simulink model "minhUpdate"  (R2022b)
settings: Solver=VariableStepAuto  StartTime=0.0  StopTime=100  RelTol=1e-3  AbsTol=1e-3  EnableMultiTasking=on
undefined symbols (not defined in the file): h, km, m, s, smiData, X, Y, Z
libraries: sm_lib x316, aerolibconvert2 x25, nesl_utility x22, simulink_extras x9, autolibshared x5, simulink x2, vehdynlibsteering x1
(part 2 of 8)

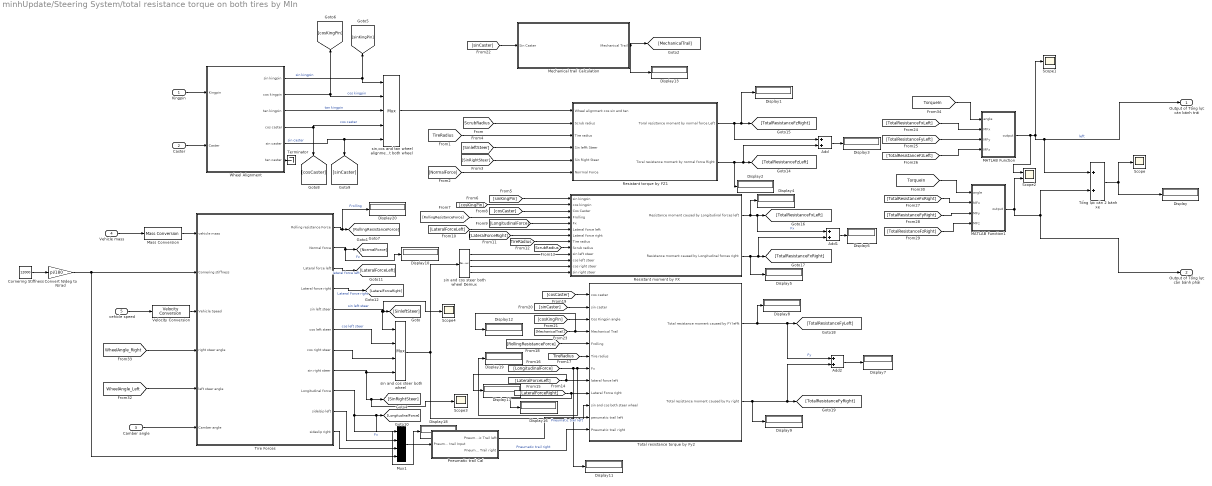
== system minhUpdate/Steering System/total resistance torque on both tires by MIn ==
  Kingpin : Inport
  Caster : Inport  Port=2
  Camber angle : Inport  Port=3
  Vehicle mass : Inport  Port=4
  "vehicle speed " : Inport  Port=5
  Add : Sum
  Add1 : Sum
  Add2 : Sum
  Convert N/deg to N/rad : Gain  Gain=pi/180
  Cornering Stiffness : Constant  Value=12000
  Display{,1..13,16..20} (19 alike) : Display
  MATLAB Function : MATLAB Function  TreatAsAtomicUnit=on
  MATLAB Function1 : MATLAB Function  TreatAsAtomicUnit=on
  Mass Conversion : aerolibconvert2/Mass Conversion  IU=kg  OU=kg
  "Mechanical trail Calculation " : Subsystem
  Mux1 : Mux
  Pneumatic trail Cal : Subsystem
  Resistant moment by FX : Subsystem
  Resistant torque by FZ1 : Subsystem
  Scope{,1,3..4} (4 alike) : Scope
  Scope2 : Scope  NumInputPorts=2
  Terminator : Terminator
  Tire Forces : Subsystem
  Total resistance torque by Fy2 : Subsystem
  Tổng lực cản 2 bánh xe : Sum
  Velocity Conversion : aerolibconvert2/Velocity Conversion  IU=km/h  OU=m/s
  Wheel Alignment : Subsystem
  sin and cos steer both wheel : Mux
  sin and cos steer both wheel Demux : Demux
  sin,cos and tan wheel alignment both wheel : Mux  Inputs=5
  Output of Tổng lực cản bánh trái : Outport
  Output of Tổng lực cản bánh phải : Outport  Port=2
  wires:
  Kingpin/1 -> Wheel Alignment/1(Kingpin)
  Wheel Alignment/6(tan caster) -> Terminator/1
  Vehicle mass/1 -> Mass Conversion/1
  Mass Conversion/1 -> Tire Forces/1(vehicle mass)
  Cornering Stiffness/1 -> Convert N/deg to N/rad/1
  Caster/1 -> Wheel Alignment/2(Caster)
  "vehicle speed "/1 -> Velocity Conversion/1
  [WheelAngle_Right] -> Tire Forces/4("right steer angle ")
  [WheelAngle_Left] -> Tire Forces/5("left steer angle ")
  Velocity Conversion/1 -> Tire Forces/3(Vehicle Speed)
  Tire Forces/11(sideslip right) -> Mux1/3
  Tire Forces/10(sidelsip left) -> Mux1/2
  Tire Forces/9(Longitudinal force) -> Mux1/1, Display18/1, [LongitudinalForce]  "Fx"
  Mux1/1 -> Pneumatic trail Cal/1(Pneumatic trail Input)
  Pneumatic trail Cal/2(Pneumatic Trail right) -> Total resistance torque by Fy2/12(Pneumatic trail right)  "Pneumatic trail right"
  Pneumatic trail Cal/1(Pneumatic Trail left) -> Total resistance torque by Fy2/11(penumatic trail left)  "Pneumatic trail left"
  Tire Forces/5(sin left steer) -> sin and cos steer both wheel/1, Scope4/1, [SinleftSteer]  "sin left steer"
  Tire Forces/6(cos left steer) -> sin and cos steer both wheel/2  "cos left steer"
  Tire Forces/7(cos right steer) -> sin and cos steer both wheel/3
  Tire Forces/8(sin right steer) -> Scope3/1, [SinRightSteer], sin and cos steer both wheel/4
  sin and cos steer both wheel/1 -> Total resistance torque by Fy2/10(sin and cos both steer wheel), sin and cos steer both wheel Demux/1
  Wheel Alignment/1(sin kingpin) -> sin,cos and tan wheel alignment both wheel/1, [sinKingPin]  "sin kingpin"
  Wheel Alignment/2(cos kingpin) -> [cosKingPin], sin,cos and tan wheel alignment both wheel/2  "cos kingpin"
  Wheel Alignment/3(tan kingpin) -> sin,cos and tan wheel alignment both wheel/3  "tan kingpin"
  Wheel Alignment/4(cos caster) -> sin,cos and tan wheel alignment both wheel/4, [cosCaster]  "cos caster"
  Wheel Alignment/5(sin caster) -> [sinCaster], sin,cos and tan wheel alignment both wheel/5  "sin caster"
  sin,cos and tan wheel alignment both wheel/1 -> Resistant torque by FZ1/1("Wheel alignment cos sin and tan ")
  Tire Forces/2(Normal force) -> Display10/1, [NormalForce]  "Fz"
  [ScrubRadius] -> Resistant torque by FZ1/2(Scrub radius)
  [TireRadius] -> Resistant torque by FZ1/3(Tire radius)
  [sinKingPin] -> Resistant moment by FX/1(sin kingpin)
  [cosKingPin] -> Resistant moment by FX/2(cos kingpin)
  Tire Forces/1(Rolling resistance Force) -> Display20/1, [RollingResistanceForce]  "Frolling"
  [RollingResistanceForce] -> Resistant moment by FX/4(Frolling)
  [cosCaster] -> Resistant moment by FX/3(Cos Caster)
  [LongitudinalForce] -> Resistant moment by FX/5(Fx)
  Tire Forces/3(Lateral force left) -> [LateralForceLeft]  "lateral force left"
  Tire Forces/4(Lateral force right) -> [LateralForceRight]  "Lateral Force right"
  [LateralForceLeft] -> Resistant moment by FX/6(Lateral force left)
  [LateralForceRight] -> Resistant moment by FX/7(Lateral force right)
  [TireRadius] -> Resistant moment by FX/8(Tire radius)
  [ScrubRadius] -> Resistant moment by FX/9(Scrub radius)
  [LateralForceRight] -> Display16/1, Total resistance torque by Fy2/9(Lateral Force right)
  [TireRadius] -> Total resistance torque by Fy2/6(Tire radius)
  [RollingResistanceForce] -> Total resistance torque by Fy2/5(Frolling)
  [cosCaster] -> Total resistance torque by Fy2/1(cos caster)
  sin and cos steer both wheel Demux/1 -> Resistant moment by FX/10(sin left steer)
  sin and cos steer both wheel Demux/2 -> Resistant moment by FX/11(cos left steer)
  sin and cos steer both wheel Demux/3 -> Resistant moment by FX/12(cos right steer)
  sin and cos steer both wheel Demux/4 -> Resistant moment by FX/13(sin right steer)
  Resistant moment by FX/1(Resistance moment caused by Longitudinal forces left) -> Display4/1, Add1/1, [TotalResistanceFxLeft]  "Fx"
  Resistant moment by FX/2(Resistance moment caused by Longitudinal forces right) -> Display5/1, Add1/2, [TotalResistanceFxRight]
  Total resistance torque by Fy2/2(Total resistance moment caused by Fy right) -> Display9/1, Add2/2, [TotalResistanceFyRight]
  Total resistance torque by Fy2/1("Total resistance moment caused by FY lefft ") -> Display8/1, Add2/1, [TotalResistanceFyLeft]  "Fy"
  [TotalResistanceFxLeft] -> MATLAB Function/2(MFx)
  [TotalResistanceFyLeft] -> MATLAB Function/3(MFy)
  [TotalResistanceFzLeft] -> MATLAB Function/4(MFz)
  [TotalResistanceFxRight] -> MATLAB Function1/2(MFx)
  [TotalResistanceFyRight] -> MATLAB Function1/3(MFy)
  [TotalResistanceFzRight] -> MATLAB Function1/4(MFz)
  Tổng lực cản 2 bánh xe/1 -> Scope/1, Display/1
  Convert N/deg to N/rad/1 -> Mux1/4, Tire Forces/2(Cornering stiffness)
  [sinCaster] -> Total resistance torque by Fy2/2(sin caster)
  [cosKingPin] -> Total resistance torque by Fy2/3(Cos Kingpin angle)
  [MechanicalTrail] -> Display12/1, Total resistance torque by Fy2/4(Mechanical Trail)
  [LongitudinalForce] -> Display19/1, Total resistance torque by Fy2/7(Fx), Display11/1
  [LateralForceLeft] -> Display17/1, Total resistance torque by Fy2/8(lateral force left)
  [SinleftSteer] -> Resistant torque by FZ1/4(Sin lefft Steer)
  [SinRightSteer] -> Resistant torque by FZ1/5(Sin Right Steer)
  [NormalForce] -> Resistant torque by FZ1/6(Norrmal Force)
  Resistant torque by FZ1/1(Toral resistance moment by normal force Left) -> Add/1, Display1/1, [TotalResistanceFzRight]
  Resistant torque by FZ1/2(Toral resistance moment by normal force Right) -> Display2/1, Add/2, [TotalResistanceFzLeft]
  Add/1 -> Display3/1
  Add1/1 -> Display6/1
  Add2/1 -> Display7/1
  "Mechanical trail Calculation "/1(Mechanical Trail) -> [MechanicalTrail], Display13/1
  [sinCaster] -> "Mechanical trail Calculation "/1(Sin Caster)
  Camber angle/1 -> Tire Forces/6(Camber angle)
  MATLAB Function/1(output) -> Scope2/1, Output of Tổng lực cản bánh trái/1, Tổng lực cản 2 bánh xe/1, Scope1/1  "left"
  [TorqueIn] -> MATLAB Function/1(angle)
  MATLAB Function1/1(output) -> Output of Tổng lực cản bánh phải/1, Tổng lực cản 2 bánh xe/2, Scope2/2
  [TorqueIn] -> MATLAB Function1/1(angle)

== system minhUpdate/total resistance torque on both tires by MIn/Mechanical trail Calculation  ==
  Sin Caster : Inport
  Display{,1..3} (4 alike) : Display
  Divide2 : Product  Inputs=**
  Scrub radius and Tire radius : Subsystem
  Mechanical Trail : Outport
  tag scope: ScrubRadius=global, TireRadius=global
  wires:
  Scrub radius and Tire radius/2(tire radius) -> Divide2/1, Display1/1, [TireRadius]  "Tire radius"
  Sin Caster/1 -> Display2/1, Divide2/2
  Divide2/1 -> Display3/1, Mechanical Trail/1  "Mechanical Trail"
  Scrub radius and Tire radius/1(scrub radius) -> [ScrubRadius], Display/1  "Scub radius"

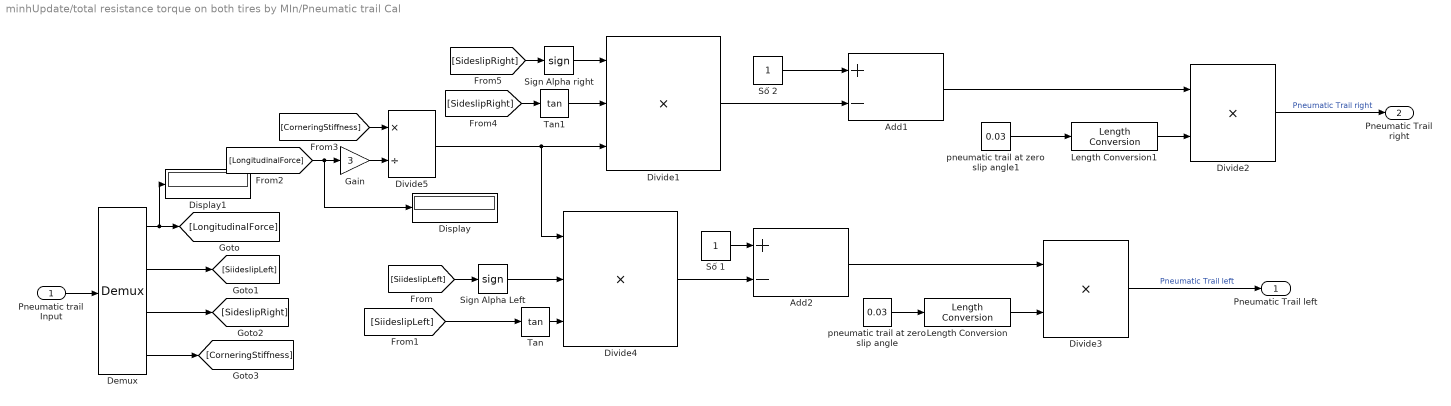
== system minhUpdate/total resistance torque on both tires by MIn/Pneumatic trail Cal ==
  Pneumatic trail Input : Inport
  Add1 : Sum  Inputs=+-
  Add2 : Sum  Inputs=+-
  Demux : Demux
  Display : Display
  Display1 : Display
  Divide1 : Product  Inputs=***
  Divide2 : Product  Inputs=**
  Divide3 : Product  Inputs=**
  Divide4 : Product  Inputs=***
  Divide5 : Product  Inputs=*/
  Gain : Gain  Gain=3
  Length Conversion : aerolibconvert2/Length Conversion  IU=m  OU=m
  Length Conversion1 : aerolibconvert2/Length Conversion  IU=m  OU=m
  Sign Alpha Left : Signum
  Sign Alpha right : Signum
  Số 1 : Constant
  Số 2 : Constant
  Tan : Trigonometry  Operator=tan
  Tan1 : Trigonometry  Operator=tan
  pneumatic trail at zero slip angle : Constant  Value=0.03
  pneumatic trail at zero slip angle1 : Constant  Value=0.03
  Pneumatic Trail left : Outport
  Pneumatic Trail right : Outport  Port=2
  wires:
  Pneumatic trail Input/1 -> Demux/1
  Divide2/1 -> Pneumatic Trail right/1  "Pneumatic Trail right"
  Length Conversion1/1 -> Divide2/2
  Add1/1 -> Divide2/1
  pneumatic trail at zero slip angle1/1 -> Length Conversion1/1
  Số 2/1 -> Add1/1
  Divide1/1 -> Add1/2
  Tan1/1 -> Divide1/2
  Sign Alpha right/1 -> Divide1/1
  Length Conversion/1 -> Divide3/2
  Divide3/1 -> Pneumatic Trail left/1  "Pneumatic Trail left"
  Add2/1 -> Divide3/1
  Gain/1 -> Divide5/2
  pneumatic trail at zero slip angle/1 -> Length Conversion/1
  Tan/1 -> Divide4/3
  Divide5/1 -> Divide4/1, Divide1/3
  Divide4/1 -> Add2/2
  Số 1/1 -> Add2/1
  Sign Alpha Left/1 -> Divide4/2
  Demux/1 -> Display1/1, [LongitudinalForce]
  Demux/2 -> [SiideslipLeft]
  Demux/3 -> [SideslipRight]
  Demux/4 -> [CorneringStiffness]
  [SiideslipLeft] -> Sign Alpha Left/1
  [SiideslipLeft] -> Tan/1
  [SideslipRight] -> Sign Alpha right/1
  [SideslipRight] -> Tan1/1
  [CorneringStiffness] -> Divide5/1
  [LongitudinalForce] -> Display/1, Gain/1

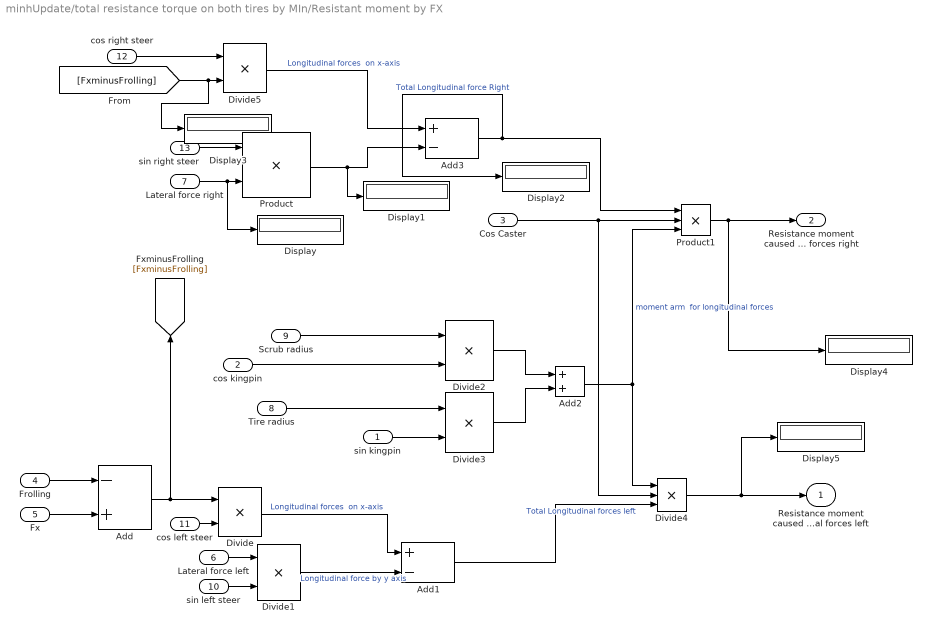
== system minhUpdate/total resistance torque on both tires by MIn/Resistant moment by FX ==
  sin kingpin : Inport
  cos kingpin : Inport  Port=2
  Cos Caster : Inport  Port=3
  Frolling : Inport  Port=4
  Fx : Inport  Port=5
  Lateral force left : Inport  Port=6
  Lateral force right : Inport  Port=7
  Tire radius : Inport  Port=8
  Scrub radius : Inport  Port=9
  sin left steer : Inport  Port=10
  cos left steer : Inport  Port=11
  cos right steer : Inport  Port=12
  sin right steer : Inport  Port=13
  Add : Sum  Inputs=-+
  Add1 : Sum  Inputs=+-
  Add2 : Sum
  Add3 : Sum  Inputs=+-
  Display{,1..5} (6 alike) : Display
  Divide{,1..3,5} (5 alike) : Product  Inputs=**
  Divide4 : Product  Inputs=***
  Product : Product
  Product1 : Product  Inputs=3
  Resistance moment caused by Longitudinal forces left : Outport
  Resistance moment caused by Longitudinal forces right : Outport  Port=2
  wires:
  Scrub radius/1 -> Divide2/1
  Divide/1 -> Add1/1  "Longitudinal forces  on x-axis"
  Divide1/1 -> Add1/2  "Longitudinal force by y axis"
  Lateral force left/1 -> Divide1/1
  Add/1 -> [FxminusFrolling], Divide/1
  Add2/1 -> Divide4/1, Product1/3  "moment arm  for longitudinal forces"
  Divide2/1 -> Add2/1
  Tire radius/1 -> Divide3/1
  Divide3/1 -> Add2/2
  cos kingpin/1 -> Divide2/2
  cos left steer/1 -> Divide/2
  sin left steer/1 -> Divide1/2
  Fx/1 -> Add/2
  Frolling/1 -> Add/1
  sin kingpin/1 -> Divide3/2
  Lateral force right/1 -> Display/1, Product/2
  sin right steer/1 -> Product/1
  Product/1 -> Display1/1, Add3/2
  cos right steer/1 -> Divide5/1
  Divide5/1 -> Add3/1  "Longitudinal forces  on x-axis"
  Add3/1 -> Display2/1, Product1/1  "Total Longitudinal force Right"
  Divide4/1 -> Display5/1, Resistance moment caused by Longitudinal forces left/1
  Cos Caster/1 -> Product1/2, Divide4/2
  Product1/1 -> Resistance moment caused by Longitudinal forces right/1, Display4/1
  [FxminusFrolling] -> Display3/1, Divide5/2
  Add1/1 -> Divide4/3  "Total Longitudinal forces left"

== system minhUpdate/total resistance torque on both tires by MIn/Resistant torque by FZ1 ==
  "Wheel alignment cos sin and tan " : Inport
  Scrub radius : Inport  Port=2
  Tire radius : Inport  Port=3
  Sin lefft Steer : Inport  Port=4
  Sin Right Steer : Inport  Port=5
  Norrmal Force : Inport  Port=6
  Add : Sum
  Demux : Demux  Outputs=5
  Display{,1..4} (5 alike) : Display
  Divide{,1..3} (4 alike) : Product  Inputs=**
  Terminator : Terminator
  Total Normal force Right : Product  Inputs=****
  Total Normal force left : Product  Inputs=****
  Toral resistance moment by normal force Left : Outport
  Toral resistance moment by normal force Right : Outport  Port=2
  wires:
  Tire radius/1 -> Divide/1
  Scrub radius/1 -> Add/1
  Total Normal force left/1 -> Divide2/2, Display1/1  "Normal force left"
  Divide1/1 -> Divide3/1, Divide2/1  "moment arm of Fz"
  Divide/1 -> Add/2
  Add/1 -> Divide1/1
  Sin lefft Steer/1 -> Display2/1, Total Normal force left/3
  Demux/3 -> Divide/2  "tan kingpin"
  Divide2/1 -> Toral resistance moment by normal force Left/1
  Demux/5 -> Terminator/1
  "Wheel alignment cos sin and tan "/1 -> Demux/1
  Sin Right Steer/1 -> Total Normal force Right/3
  Norrmal Force/1 -> Display/1, Total Normal force left/4, Total Normal force Right/4
  Total Normal force Right/1 -> Divide3/2  "Normal force right"
  Divide3/1 -> Toral resistance moment by normal force Right/1
  Demux/1 -> [sinKingpin]  "sin kingppin"
  Demux/2 -> [cosKingpin]  "cos kingpin"
  Demux/4 -> [cosCaster]  "cos caster"
  [cosKingpin] -> Divide1/2
  [cosCaster] -> Total Normal force Right/2
  [sinKingpin] -> Total Normal force Right/1
  [sinKingpin] -> Display3/1, Total Normal force left/1
  [cosCaster] -> Display4/1, Total Normal force left/2

== system minhUpdate/total resistance torque on both tires by MIn/Tire Forces ==
  vehicle mass : Inport
  Cornering stiffness : Inport  Port=2
  Vehicle Speed : Inport  Port=3
  "right steer angle " : Inport  Port=4
  "left steer angle " : Inport  Port=5
  Camber angle : Inport  Port=6
  Add : Sum
  Add1 : Sum
  Cos : Trigonometry  Operator=cos
  Cos1 : Trigonometry  Operator=cos
  Display{,1..4} (5 alike) : Display
  Lateral Force Area : Subsystem
  Mass Conversion : aerolibconvert2/Mass Conversion  IU=kg  OU=kg
  Multiply : Gain  Gain=130
  Normal and Longitudinal force Area : Subsystem
  Rolling Resistance area : Subsystem
  Sin1 : Trigonometry
  Sin2 : Trigonometry
  Rolling resistance Force : Outport
  Normal force : Outport  Port=2
  Lateral force left : Outport  Port=3
  Lateral force right : Outport  Port=4
  sin left steer : Outport  Port=5
  cos left steer : Outport  Port=6
  cos right steer : Outport  Port=7
  sin right steer : Outport  Port=8
  Longitudinal force : Outport  Port=9
  sidelsip left : Outport  Port=10
  sideslip right : Outport  Port=11
  wires:
  Lateral Force Area/4(Right Steer angle) -> Sin2/1, Cos1/1
  vehicle mass/1 -> Display/1, Mass Conversion/1
  Sin2/1 -> sin right steer/1  "sin right  steer"
  Cos1/1 -> cos right steer/1  "cos right steer"
  Normal and Longitudinal force Area/1(Longitudinal force) -> Longitudinal force/1
  Normal and Longitudinal force Area/2(Normal force) -> Normal force/1
  Rolling Resistance area/1(rolling resitance force) -> Rolling resistance Force/1  "Rolling resistance Force"
  Lateral Force Area/5(sideslip left) -> sidelsip left/1
  Lateral Force Area/6("sideslip right ") -> sideslip right/1
  Cornering stiffness/1 -> Lateral Force Area/1("Cornering Stiffness ")
  Mass Conversion/1 -> Display1/1, Normal and Longitudinal force Area/1(vehicle mass), Display2/1, Rolling Resistance area/1(vehicle mass)
  Vehicle Speed/1 -> Lateral Force Area/2(Vehicle Speed)
  "left steer angle "/1 -> Lateral Force Area/4(Steering angle from left)
  "right steer angle "/1 -> Lateral Force Area/3(Steering angle right)
  Lateral Force Area/3(Left steer angle) -> Sin1/1, Cos/1
  Sin1/1 -> sin left steer/1  "sin left  steer"
  Cos/1 -> cos left steer/1  "cos left steer"
  Camber angle/1 -> Multiply/1
  Multiply/1 -> Add1/1, Add/1
  Lateral Force Area/1(Lateral force left(N)) -> Add/2
  Lateral Force Area/2("Lateral force right(N)  ") -> Add1/2
  Add1/1 -> Display4/1, Lateral force right/1
  Add/1 -> Display3/1, Lateral force left/1

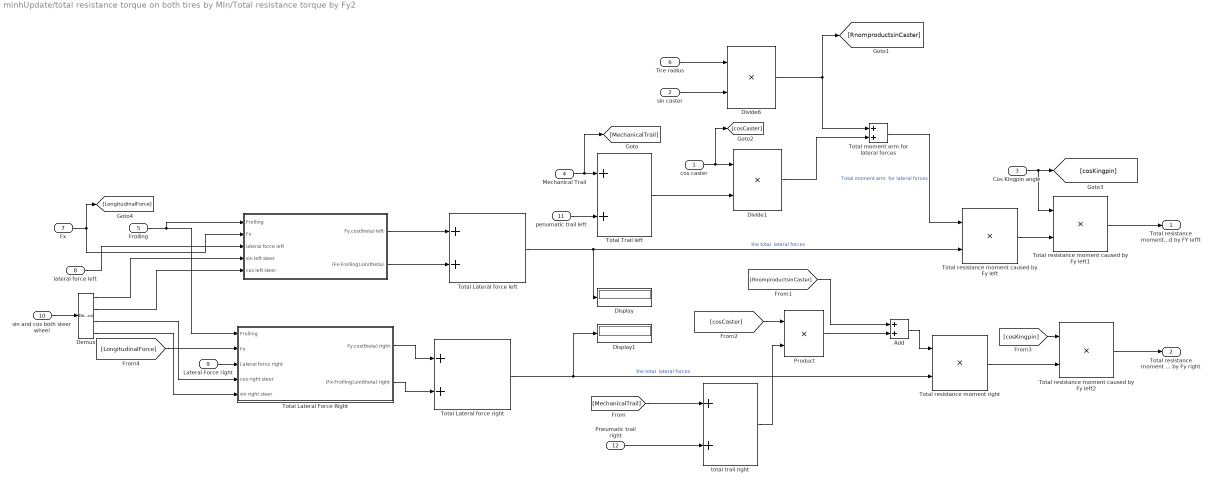
== system minhUpdate/total resistance torque on both tires by MIn/Total resistance torque by Fy2 ==
  cos caster : Inport
  sin caster : Inport  Port=2
  Cos Kingpin angle : Inport  Port=3
  Mechanical Trail : Inport  Port=4
  Frolling : Inport  Port=5
  Tire radius : Inport  Port=6
  Fx : Inport  Port=7
  lateral force left : Inport  Port=8
  Lateral Force right : Inport  Port=9
  sin and cos both steer wheel : Inport  Port=10
  penumatic trail left : Inport  Port=11
  Pneumatic trail right : Inport  Port=12
  " " : Subsystem
  " Total Lateral Force Right " : Subsystem
  Add : Sum
  Demux : Demux
  Display : Display
  Display1 : Display
  Divide1 : Product  Inputs=**
  Divide6 : Product  Inputs=**
  Product : Product
  Total Lateral force left : Sum
  Total Lateral force right : Sum
  Total Trail left : Sum
  Total moment arm for lateral forces : Sum
  Total resistance moment caused by Fy left : Product  Inputs=**
  Total resistance moment caused by Fy left1 : Product  Inputs=**
  Total resistance moment caused by Fy left2 : Product  Inputs=**
  Total resistance moment right : Product  Inputs=**
  total trail right : Sum
  "Total resistance moment caused by FY lefft " : Outport
  Total resistance moment caused by Fy right : Outport  Port=2
  wires:
  cos caster/1 -> [cosCaster], Divide1/1
  Divide6/1 -> [RnomproductsinCaster], Total moment arm for lateral forces/1
  Total moment arm for lateral forces/1 -> Total resistance moment caused by Fy left/1  "Total moment arm  for lateral forces"
  Total Lateral force left/1 -> Display/1, Total resistance moment caused by Fy left/2  "the total  lateral forces"
  Divide1/1 -> Total moment arm for lateral forces/2
  " "/1(Fy.cos(theta) left) -> Total Lateral force left/1
  Total Trail left/1 -> Divide1/2
  " "/2((Fx-Frolling).sin(theta)) -> Total Lateral force left/2
  penumatic trail left/1 -> Total Trail left/2
  Tire radius/1 -> Divide6/1
  sin caster/1 -> Divide6/2
  Frolling/1 -> " Total Lateral Force Right "/1(Frolling), " "/1(Frolling)
  lateral force left/1 -> " "/3(lateral force left)
  Mechanical Trail/1 -> [MechanicalTrail], Total Trail left/1
  Lateral Force right/1 -> " Total Lateral Force Right "/3(Lateral force right)
  Demux/3 -> " Total Lateral Force Right "/4(cos right steer)
  Demux/4 -> " Total Lateral Force Right "/5(sin right steer)
  " Total Lateral Force Right "/1(Fy.cos(theta) right) -> Total Lateral force right/1
  " Total Lateral Force Right "/2((Fx-Frolling).sin(theta) right) -> Total Lateral force right/2
  Total Lateral force right/1 -> Display1/1, Total resistance moment right/2  "the total  lateral forces"
  Cos Kingpin angle/1 -> [cosKingpin], Total resistance moment caused by Fy left1/1
  Total resistance moment caused by Fy left/1 -> Total resistance moment caused by Fy left1/2
  Total resistance moment caused by Fy left1/1 -> "Total resistance moment caused by FY lefft "/1
  Total resistance moment right/1 -> Total resistance moment caused by Fy left2/2
  Total resistance moment caused by Fy left2/1 -> Total resistance moment caused by Fy right/1
  Pneumatic trail right/1 -> total trail right/2
  total trail right/1 -> Product/2
  Product/1 -> Add/2
  Add/1 -> Total resistance moment right/1
  Demux/1 -> " "/4(sin left steer)
  Demux/2 -> " "/5(cos left steer)
  sin and cos both steer wheel/1 -> Demux/1
  [MechanicalTrail] -> total trail right/1
  [RnomproductsinCaster] -> Add/1
  [cosCaster] -> Product/1
  [cosKingpin] -> Total resistance moment caused by Fy left2/1
  Fx/1 -> " "/2(Fx), [LongitudinalForce]
  [LongitudinalForce] -> " Total Lateral Force Right "/2(Fx)

== system minhUpdate/total resistance torque on both tires by MIn/Wheel Alignment ==
  Kingpin : Inport
  Caster : Inport  Port=2
  Cos : Trigonometry  Operator=cos
  Cos1 : Trigonometry  Operator=cos
  Degrees to Radians : simulink_extras/Transformations/Degrees to Radians
  Degrees to Radians1 : simulink_extras/Transformations/Degrees to Radians
  Display : Display
  Sin : Trigonometry
  Sin1 : Trigonometry
  Tan : Trigonometry  Operator=tan
  Tan1 : Trigonometry  Operator=tan
  sin kingpin : Outport
  cos kingpin : Outport  Port=2
  tan kingpin : Outport  Port=3
  cos caster : Outport  Port=4
  sin caster : Outport  Port=5
  tan caster : Outport  Port=6
  wires:
  Sin1/1 -> sin caster/1
  Degrees to Radians1/1 -> Tan1/1, Sin1/1, Cos1/1
  Sin/1 -> sin kingpin/1
  Caster/1 -> Degrees to Radians1/1
  Cos1/1 -> cos caster/1
  Cos/1 -> cos kingpin/1
  Degrees to Radians/1 -> Tan/1, Sin/1, Cos/1
  Kingpin/1 -> Degrees to Radians/1
  Tan/1 -> Display/1, tan kingpin/1
  Tan1/1 -> tan caster/1

== system minhUpdate/Steering System/Chassis + Rack/Rack Case + Chassis ==
  PS-Simulink Converter : nesl_utility/PS-Simulink Converter  PhysicalDomain=network_engine_domain  SubClassName=ps_output  LeftPortType=input  RightPortType=output  PseudoPeriodic=off  Frequencies=[]  VectorFormat=1-D array  Unit=inherit  AffineConversion=off
  PS-Simulink Converter1 : nesl_utility/PS-Simulink Converter  PhysicalDomain=network_engine_domain  SubClassName=ps_output  LeftPortType=input  RightPortType=output  PseudoPeriodic=off  Frequencies=[]  VectorFormat=1-D array  Unit=inherit  AffineConversion=off
  Parallel : sm_lib/Constraints/Angle Constraint  ConstraintType=Parallel  Angle=45  AngleUnits=deg  SenseSignedTorqueMagnitude=off  SenseTorque=off  SenseForce=off  WrenchDir=FollowerOnBase  WrenchFrame=BaseFrame
  Parallel1 : sm_lib/Constraints/Angle Constraint  ConstraintType=Parallel  Angle=45  AngleUnits=deg  SenseSignedTorqueMagnitude=off  SenseTorque=off  SenseForce=off  WrenchDir=FollowerOnBase  WrenchFrame=BaseFrame
  Prismatic Joint : sm_lib/Joints/Prismatic Joint  JointMode=Normal  SenseConstraintForce=off  SenseConstraintForceX=off  SenseConstraintForceY=off  SenseConstraintForceZ=off  SenseConstraintTorque=off  SenseConstraintTorqueX=off  SenseConstraintTorqueY=off  SenseConstraintTorqueZ=off  SenseTotalForce=off  SenseTotalForceX=off  SenseTotalForceY=off  SenseTotalForceZ=off  SenseTotalTorque=off  SenseTotalTorqueX=off  SenseTotalTorqueY=off  SenseTotalTorqueZ=off  CompositeWrenchDir=FollowerOnBase  CompositeWrenchFrame=BaseFrame  EquilibriumPosition=0  EquilibriumPositionUnits=m  SpringStiffness=0  SpringStiffnessUnits=N/m  DampingCoefficient=0  DampingCoefficientUnits=N/(m/s)  TorqueActuationMode=NoTorque  MotionActuationMode=ComputedMotion  SensePosition=off  SenseVelocity=off  SenseAcceleration=off  SenseTorqueForce=off  SenseLowerLimitTorqueForce=off  SenseUpperLimitTorqueForce=off  LowerLimitSpecify=off  LowerLimitBound=-1  LowerLimitBoundUnits=m  LowerLimitStiffness=1e6  LowerLimitStiffnessUnits=N/m  LowerLimitDamping=1e3  LowerLimitDampingUnits=N/(m/s)  LowerLimitTransitionRegionWidth=1e-4  LowerLimitTransitionRegionWidthUnits=m  UpperLimitSpecify=off  UpperLimitBound=1  UpperLimitBoundUnits=m  UpperLimitStiffness=1e6  UpperLimitStiffnessUnits=N/m  UpperLimitDamping=1e3  UpperLimitDampingUnits=N/(m/s)  UpperLimitTransitionRegionWidth=1e-4  UpperLimitTransitionRegionWidthUnits=m  PositionTargetSpecify=off  PositionTargetPriority=High  PositionTargetValue=0  PositionTargetValueUnits=m  VelocityTargetSpecify=off  VelocityTargetPriority=High  VelocityTargetValue=0  VelocityTargetValueUnits=m/s
  Rack_housing_1_RIGID : Subsystem
  Revolute Joint : sm_lib/Joints/Revolute Joint  JointMode=Normal  SenseConstraintForce=off  SenseConstraintForceX=off  SenseConstraintForceY=off  SenseConstraintForceZ=off  SenseConstraintTorque=off  SenseConstraintTorqueX=off  SenseConstraintTorqueY=off  SenseConstraintTorqueZ=off  SenseTotalForce=off  SenseTotalForceX=off  SenseTotalForceY=off  SenseTotalForceZ=off  SenseTotalTorque=off  SenseTotalTorqueX=off  SenseTotalTorqueY=off  SenseTotalTorqueZ=off  CompositeWrenchDir=FollowerOnBase  CompositeWrenchFrame=BaseFrame  EquilibriumPosition=0  EquilibriumPositionUnits=deg  SpringStiffness=0  SpringStiffnessUnits=N*m/rad  DampingCoefficient=8  DampingCoefficientUnits=N*m/(rad/s)  TorqueActuationMode=NoTorque  MotionActuationMode=ComputedMotion  SensePosition=on  SenseVelocity=on  SenseAcceleration=off  SenseTorqueForce=off  SenseLowerLimitTorqueForce=off  SenseUpperLimitTorqueForce=off  LowerLimitSpecify=off  LowerLimitBound=-90  LowerLimitBoundUnits=deg  LowerLimitStiffness=1e4  LowerLimitStiffnessUnits=N*m/deg  LowerLimitDamping=10  LowerLimitDampingUnits=N*m/(deg/s)  LowerLimitTransitionRegionWidth=0.1  LowerLimitTransitionRegionWidthUnits=deg  UpperLimitSpecify=off  UpperLimitBound=90  UpperLimitBoundUnits=deg  UpperLimitStiffness=1e4  UpperLimitStiffnessUnits=N*m/deg  UpperLimitDamping=10  UpperLimitDampingUnits=N*m/(deg/s)  UpperLimitTransitionRegionWidth=0.1  UpperLimitTransitionRegionWidthUnits=deg  PositionTargetSpecify=off  PositionTargetPriority=High  PositionTargetValue=0  PositionTargetValueUnits=deg  VelocityTargetSpecify=on  VelocityTargetPriority=High  VelocityTargetValue=0  VelocityTargetValueUnits=deg/s
  Revolute4 : sm_lib/Joints/Revolute Joint  JointMode=Normal  SenseConstraintForce=off  SenseConstraintForceX=off  SenseConstraintForceY=off  SenseConstraintForceZ=off  SenseConstraintTorque=off  SenseConstraintTorqueX=off  SenseConstraintTorqueY=off  SenseConstraintTorqueZ=off  SenseTotalForce=off  SenseTotalForceX=off  SenseTotalForceY=off  SenseTotalForceZ=off  SenseTotalTorque=off  SenseTotalTorqueX=off  SenseTotalTorqueY=off  SenseTotalTorqueZ=off  CompositeWrenchDir=FollowerOnBase  CompositeWrenchFrame=BaseFrame  EquilibriumPosition=0  EquilibriumPositionUnits=deg  SpringStiffness=0  SpringStiffnessUnits=N*m/deg  DampingCoefficient=0  DampingCoefficientUnits=N*m/(deg/s)  TorqueActuationMode=NoTorque  MotionActuationMode=ComputedMotion  SensePosition=off  SenseVelocity=off  SenseAcceleration=off  SenseTorqueForce=off  SenseLowerLimitTorqueForce=off  SenseUpperLimitTorqueForce=off  LowerLimitSpecify=off  LowerLimitBound=-90  LowerLimitBoundUnits=deg  LowerLimitStiffness=1e4  LowerLimitStiffnessUnits=N*m/deg  LowerLimitDamping=10  LowerLimitDampingUnits=N*m/(deg/s)  LowerLimitTransitionRegionWidth=0.1  LowerLimitTransitionRegionWidthUnits=deg  UpperLimitSpecify=off  UpperLimitBound=90  UpperLimitBoundUnits=deg  UpperLimitStiffness=1e4  UpperLimitStiffnessUnits=N*m/deg  UpperLimitDamping=10  UpperLimitDampingUnits=N*m/(deg/s)  UpperLimitTransitionRegionWidth=0.1  UpperLimitTransitionRegionWidthUnits=deg  PositionTargetSpecify=on  PositionTargetPriority=Low  PositionTargetValue=smiData.RevoluteJoint(5).Rz.Pos  PositionTargetValueUnits=deg  VelocityTargetSpecify=off  VelocityTargetPriority=High  VelocityTargetValue=0  VelocityTargetValueUnits=deg/s
  Revolute5 : sm_lib/Joints/Revolute Joint  JointMode=Normal  SenseConstraintForce=off  SenseConstraintForceX=off  SenseConstraintForceY=off  SenseConstraintForceZ=off  SenseConstraintTorque=off  SenseConstraintTorqueX=off  SenseConstraintTorqueY=off  SenseConstraintTorqueZ=off  SenseTotalForce=off  SenseTotalForceX=off  SenseTotalForceY=off  SenseTotalForceZ=off  SenseTotalTorque=off  SenseTotalTorqueX=off  SenseTotalTorqueY=off  SenseTotalTorqueZ=off  CompositeWrenchDir=FollowerOnBase  CompositeWrenchFrame=BaseFrame  EquilibriumPosition=0  EquilibriumPositionUnits=deg  SpringStiffness=0  SpringStiffnessUnits=N*m/deg  DampingCoefficient=0  DampingCoefficientUnits=N*m/(deg/s)  TorqueActuationMode=NoTorque  MotionActuationMode=ComputedMotion  SensePosition=off  SenseVelocity=off  SenseAcceleration=off  SenseTorqueForce=off  SenseLowerLimitTorqueForce=off  SenseUpperLimitTorqueForce=off  LowerLimitSpecify=off  LowerLimitBound=-90  LowerLimitBoundUnits=deg  LowerLimitStiffness=1e4  LowerLimitStiffnessUnits=N*m/deg  LowerLimitDamping=10  LowerLimitDampingUnits=N*m/(deg/s)  LowerLimitTransitionRegionWidth=0.1  LowerLimitTransitionRegionWidthUnits=deg  UpperLimitSpecify=off  UpperLimitBound=90  UpperLimitBoundUnits=deg  UpperLimitStiffness=1e4  UpperLimitStiffnessUnits=N*m/deg  UpperLimitDamping=10  UpperLimitDampingUnits=N*m/(deg/s)  UpperLimitTransitionRegionWidth=0.1  UpperLimitTransitionRegionWidthUnits=deg  PositionTargetSpecify=on  PositionTargetPriority=Low  PositionTargetValue=smiData.RevoluteJoint(6).Rz.Pos  PositionTargetValueUnits=deg  VelocityTargetSpecify=off  VelocityTargetPriority=High  VelocityTargetValue=0  VelocityTargetValueUnits=deg/s
  Revolute6 : sm_lib/Joints/Revolute Joint  JointMode=Normal  SenseConstraintForce=off  SenseConstraintForceX=off  SenseConstraintForceY=off  SenseConstraintForceZ=off  SenseConstraintTorque=off  SenseConstraintTorqueX=off  SenseConstraintTorqueY=off  SenseConstraintTorqueZ=off  SenseTotalForce=off  SenseTotalForceX=off  SenseTotalForceY=off  SenseTotalForceZ=off  SenseTotalTorque=off  SenseTotalTorqueX=off  SenseTotalTorqueY=off  SenseTotalTorqueZ=off  CompositeWrenchDir=FollowerOnBase  CompositeWrenchFrame=BaseFrame  EquilibriumPosition=0  EquilibriumPositionUnits=deg  SpringStiffness=0  SpringStiffnessUnits=N*m/deg  DampingCoefficient=0  DampingCoefficientUnits=N*m/(deg/s)  TorqueActuationMode=NoTorque  MotionActuationMode=ComputedMotion  SensePosition=off  SenseVelocity=off  SenseAcceleration=off  SenseTorqueForce=off  SenseLowerLimitTorqueForce=off  SenseUpperLimitTorqueForce=off  LowerLimitSpecify=off  LowerLimitBound=-90  LowerLimitBoundUnits=deg  LowerLimitStiffness=1e4  LowerLimitStiffnessUnits=N*m/deg  LowerLimitDamping=10  LowerLimitDampingUnits=N*m/(deg/s)  LowerLimitTransitionRegionWidth=0.1  LowerLimitTransitionRegionWidthUnits=deg  UpperLimitSpecify=off  UpperLimitBound=90  UpperLimitBoundUnits=deg  UpperLimitStiffness=1e4  UpperLimitStiffnessUnits=N*m/deg  UpperLimitDamping=10  UpperLimitDampingUnits=N*m/(deg/s)  UpperLimitTransitionRegionWidth=0.1  UpperLimitTransitionRegionWidthUnits=deg  PositionTargetSpecify=on  PositionTargetPriority=Low  PositionTargetValue=smiData.RevoluteJoint(7).Rz.Pos  PositionTargetValueUnits=deg  VelocityTargetSpecify=off  VelocityTargetPriority=High  VelocityTargetValue=0  VelocityTargetValueUnits=deg/s
  Revolute7 : sm_lib/Joints/Revolute Joint  JointMode=Normal  SenseConstraintForce=off  SenseConstraintForceX=off  SenseConstraintForceY=off  SenseConstraintForceZ=off  SenseConstraintTorque=off  SenseConstraintTorqueX=off  SenseConstraintTorqueY=off  SenseConstraintTorqueZ=off  SenseTotalForce=off  SenseTotalForceX=off  SenseTotalForceY=off  SenseTotalForceZ=off  SenseTotalTorque=off  SenseTotalTorqueX=off  SenseTotalTorqueY=off  SenseTotalTorqueZ=off  CompositeWrenchDir=FollowerOnBase  CompositeWrenchFrame=BaseFrame  EquilibriumPosition=0  EquilibriumPositionUnits=deg  SpringStiffness=0  SpringStiffnessUnits=N*m/deg  DampingCoefficient=0  DampingCoefficientUnits=N*m/(deg/s)  TorqueActuationMode=NoTorque  MotionActuationMode=ComputedMotion  SensePosition=off  SenseVelocity=off  SenseAcceleration=off  SenseTorqueForce=off  SenseLowerLimitTorqueForce=off  SenseUpperLimitTorqueForce=off  LowerLimitSpecify=off  LowerLimitBound=-90  LowerLimitBoundUnits=deg  LowerLimitStiffness=1e4  LowerLimitStiffnessUnits=N*m/deg  LowerLimitDamping=10  LowerLimitDampingUnits=N*m/(deg/s)  LowerLimitTransitionRegionWidth=0.1  LowerLimitTransitionRegionWidthUnits=deg  UpperLimitSpecify=off  UpperLimitBound=90  UpperLimitBoundUnits=deg  UpperLimitStiffness=1e4  UpperLimitStiffnessUnits=N*m/deg  UpperLimitDamping=10  UpperLimitDampingUnits=N*m/(deg/s)  UpperLimitTransitionRegionWidth=0.1  UpperLimitTransitionRegionWidthUnits=deg  PositionTargetSpecify=on  PositionTargetPriority=Low  PositionTargetValue=smiData.RevoluteJoint(8).Rz.Pos  PositionTargetValueUnits=deg  VelocityTargetSpecify=off  VelocityTargetPriority=High  VelocityTargetValue=0  VelocityTargetValueUnits=deg/s
  Revolute8 : sm_lib/Joints/Revolute Joint  JointMode=Normal  SenseConstraintForce=off  SenseConstraintForceX=off  SenseConstraintForceY=off  SenseConstraintForceZ=off  SenseConstraintTorque=off  SenseConstraintTorqueX=off  SenseConstraintTorqueY=off  SenseConstraintTorqueZ=off  SenseTotalForce=off  SenseTotalForceX=off  SenseTotalForceY=off  SenseTotalForceZ=off  SenseTotalTorque=off  SenseTotalTorqueX=off  SenseTotalTorqueY=off  SenseTotalTorqueZ=off  CompositeWrenchDir=FollowerOnBase  CompositeWrenchFrame=BaseFrame  EquilibriumPosition=0  EquilibriumPositionUnits=deg  SpringStiffness=0  SpringStiffnessUnits=N*m/deg  DampingCoefficient=0  DampingCoefficientUnits=N*m/(deg/s)  TorqueActuationMode=NoTorque  MotionActuationMode=ComputedMotion  SensePosition=off  SenseVelocity=off  SenseAcceleration=off  SenseTorqueForce=off  SenseLowerLimitTorqueForce=off  SenseUpperLimitTorqueForce=off  LowerLimitSpecify=off  LowerLimitBound=-90  LowerLimitBoundUnits=deg  LowerLimitStiffness=1e4  LowerLimitStiffnessUnits=N*m/deg  LowerLimitDamping=10  LowerLimitDampingUnits=N*m/(deg/s)  LowerLimitTransitionRegionWidth=0.1  LowerLimitTransitionRegionWidthUnits=deg  UpperLimitSpecify=off  UpperLimitBound=90  UpperLimitBoundUnits=deg  UpperLimitStiffness=1e4  UpperLimitStiffnessUnits=N*m/deg  UpperLimitDamping=10  UpperLimitDampingUnits=N*m/(deg/s)  UpperLimitTransitionRegionWidth=0.1  UpperLimitTransitionRegionWidthUnits=deg  PositionTargetSpecify=on  PositionTargetPriority=Low  PositionTargetValue=smiData.RevoluteJoint(9).Rz.Pos  PositionTargetValueUnits=deg  VelocityTargetSpecify=off  VelocityTargetPriority=High  VelocityTargetValue=0  VelocityTargetValueUnits=deg/s
  Revolute9 : sm_lib/Joints/Revolute Joint  JointMode=Normal  SenseConstraintForce=off  SenseConstraintForceX=off  SenseConstraintForceY=off  SenseConstraintForceZ=off  SenseConstraintTorque=off  SenseConstraintTorqueX=off  SenseConstraintTorqueY=off  SenseConstraintTorqueZ=off  SenseTotalForce=off  SenseTotalForceX=off  SenseTotalForceY=off  SenseTotalForceZ=off  SenseTotalTorque=off  SenseTotalTorqueX=off  SenseTotalTorqueY=off  SenseTotalTorqueZ=off  CompositeWrenchDir=FollowerOnBase  CompositeWrenchFrame=BaseFrame  EquilibriumPosition=0  EquilibriumPositionUnits=deg  SpringStiffness=0  SpringStiffnessUnits=N*m/deg  DampingCoefficient=0  DampingCoefficientUnits=N*m/(deg/s)  TorqueActuationMode=NoTorque  MotionActuationMode=ComputedMotion  SensePosition=off  SenseVelocity=off  SenseAcceleration=off  SenseTorqueForce=off  SenseLowerLimitTorqueForce=off  SenseUpperLimitTorqueForce=off  LowerLimitSpecify=off  LowerLimitBound=-90  LowerLimitBoundUnits=deg  LowerLimitStiffness=1e4  LowerLimitStiffnessUnits=N*m/deg  LowerLimitDamping=10  LowerLimitDampingUnits=N*m/(deg/s)  LowerLimitTransitionRegionWidth=0.1  LowerLimitTransitionRegionWidthUnits=deg  UpperLimitSpecify=off  UpperLimitBound=90  UpperLimitBoundUnits=deg  UpperLimitStiffness=1e4  UpperLimitStiffnessUnits=N*m/deg  UpperLimitDamping=10  UpperLimitDampingUnits=N*m/(deg/s)  UpperLimitTransitionRegionWidth=0.1  UpperLimitTransitionRegionWidthUnits=deg  PositionTargetSpecify=off  PositionTargetPriority=High  PositionTargetValue=0  PositionTargetValueUnits=deg  VelocityTargetSpecify=off  VelocityTargetPriority=High  VelocityTargetValue=0  VelocityTargetValueUnits=deg/s
  Transform : sm_lib/Frames and Transforms/Rigid Transform  TranslationMethod=Cartesian  TranslationStandardOffset=0  TranslationLengthUnit=mm  TranslationStandardAxis=+Z  TranslationCartesianOffset=smiData.RigidTransform(47).translation  TranslationROffset=0  TranslationROffsetUnits=m  TranslationZOffset=0  TranslationZOffsetUnits=m  TranslationThetaOffset=0  TranslationThetaOffsetUnits=deg  RotationMethod=ArbitraryAxis  RotationAngleUnits=rad  RotationStandardAxis=+Z  RotationAngle=smiData.RigidTransform(47).angle  RotationArbitraryAxis=smiData.RigidTransform(47).axis  FollAlignAxisA=+X  BaseAlignAxisA=+Y  FollAlignAxisB=+Y  BaseAlignAxisB=+Z  RotationSequenceAxes=FollowerAxes  RotationSequence=XYX  RotationSequenceAngles=[0 0 0]  RotationSequenceAnglesUnits=deg  RotationMatrix=[1 0 0; 0 1 0; 0 0 1]  Quaternion=[1 0 0 0]
  extention_rod_1_RIGID : Subsystem
  extention_rod_2_RIGID : Subsystem
  extention_rod_image_1_RIGID : Subsystem
  extention_rod_image_2_RIGID : Subsystem
  lever_arm_by_Long_1_RIGID : Subsystem
  lever_arm_by_Long_2_RIGID : Subsystem
  lever_arm_mini_by_Long_1_RIGID : Subsystem
  lever_arm_mini_by_Long_2_RIGID : Subsystem
  Conn1 : PMIOPort  Side=Left
  Conn3 : PMIOPort  Port=2  Side=Left
  Conn4 : PMIOPort  Port=3  Side=Left
  Conn5 : PMIOPort  Port=4  Side=Left
  F : PMIOPort  Port=5  Side=Left
  F1 : PMIOPort  Port=6  Side=Left
  F2 : PMIOPort  Port=7  Side=Left
  Conn2 : PMIOPort  Port=8  Side=Right
  F3 : PMIOPort  Port=9  Side=Right
  Steering Wheel Angle : Outport
  Steering Wheel Velocity : Outport  Port=2
  wires:
  PS-Simulink Converter/1 -> Steering Wheel Angle/1
  PS-Simulink Converter1/1 -> Steering Wheel Velocity/1
  connections:
  Parallel/RConn1 -- extention_rod_1_RIGID/LConn1
  Revolute Joint/RConn1 -- Rack_housing_1_RIGID/LConn2
  Revolute8/LConn1 -- lever_arm_by_Long_2_RIGID/RConn1
  Parallel/LConn1 -- Rack_housing_1_RIGID/RConn2
  Parallel1/LConn1 -- Rack_housing_1_RIGID/RConn1
  F/RConn1 -- extention_rod_image_2_RIGID/LConn1
  Rack_housing_1_RIGID/LConn1 -- Transform/RConn1
  Parallel1/RConn1 -- extention_rod_2_RIGID/LConn1
  Revolute6/RConn1 -- lever_arm_mini_by_Long_1_RIGID/LConn1
  Revolute4/RConn1 -- extention_rod_1_RIGID/LConn2
  Revolute7/RConn1 -- lever_arm_by_Long_1_RIGID/LConn1
  Revolute9/RConn1 -- lever_arm_by_Long_2_RIGID/LConn1
  Revolute6/LConn1 -- lever_arm_by_Long_1_RIGID/RConn1
  Revolute7/LConn1 -- extention_rod_1_RIGID/RConn1
  Revolute5/RConn1 -- extention_rod_2_RIGID/LConn2
  Prismatic Joint/LConn1 -- Rack_housing_1_RIGID/LConn3
  Revolute9/LConn1 -- extention_rod_2_RIGID/RConn1
  Revolute8/RConn1 -- lever_arm_mini_by_Long_2_RIGID/LConn1
  Conn4/RConn1 -- Revolute4/LConn1
  extention_rod_image_1_RIGID/LConn1 -- F1/RConn1
  Prismatic Joint/RConn1 -- Conn5/RConn1
  Conn3/RConn1 -- Revolute5/LConn1
  Revolute Joint/LConn1 -- Conn2/RConn1
  lever_arm_mini_by_Long_2_RIGID/RConn1 -- F3/RConn1
  Conn1/RConn1 -- Transform/LConn1
  lever_arm_mini_by_Long_1_RIGID/RConn1 -- F2/RConn1
  PS-Simulink Converter/LConn1 -- Revolute Joint/RConn2
  PS-Simulink Converter1/LConn1 -- Revolute Joint/RConn3

== system minhUpdate/Steering System/Chassis + Rack/Rack_1_RIGID ==
  ReferenceFrame : sm_lib/Frames and Transforms/Reference Frame
  Solid : sm_lib/Body Elements/File Solid  ExtGeomFileName=Rack_Default_sldprt.STEP  UnitType=FromFile  ExtGeomFileUnits=m  StepReaderType=HEX  ExportConvexHullGeometry=off  InertiaType=Custom  Mass=smiData.Solid(7).mass  MassUnits=kg  CenterOfMass=smiData.Solid(7).CoM  CenterOfMassUnits=mm  MomentsOfInertia=smiData.Solid(7).MoI  MomentsOfInertiaUnits=kg*mm^2  ProductsOfInertia=smiData.Solid(7).PoI  ProductsOfInertiaUnits=kg*mm^2  BasedOnType=DensityFromFile  Density=1000  DensityUnits=kg/m^3  DoExposeReferenceFrame=on  SerializedFrames=<Frames/>  GraphicType=FromGeometry  MarkerShape=Sphere  MarkerSize=10  GraphicVisPropType=SimpleVisualProperties  GraphicDiffuseColor=smiData.Solid(7).color  GraphicSpecularColor=[0.5 0.5 0.5 1.0]  GraphicAmbientColor=[0.15 0.15 0.15 1.0]  GraphicEmissiveColor=[0.0 0.0 0.0 1.0]  GraphicShininess=75  GraphicOpacity=smiData.Solid(7).opacity
  Transform : sm_lib/Frames and Transforms/Rigid Transform  TranslationMethod=Cartesian  TranslationStandardOffset=0  TranslationLengthUnit=mm  TranslationStandardAxis=+Z  TranslationCartesianOffset=smiData.RigidTransform(5).translation  TranslationROffset=0  TranslationROffsetUnits=m  TranslationZOffset=0  TranslationZOffsetUnits=m  TranslationThetaOffset=0  TranslationThetaOffsetUnits=deg  RotationMethod=ArbitraryAxis  RotationAngleUnits=rad  RotationStandardAxis=+Z  RotationAngle=smiData.RigidTransform(5).angle  RotationArbitraryAxis=smiData.RigidTransform(5).axis  FollAlignAxisA=+X  BaseAlignAxisA=+Y  FollAlignAxisB=+Y  BaseAlignAxisB=+Z  RotationSequenceAxes=FollowerAxes  RotationSequence=XYX  RotationSequenceAngles=[0 0 0]  RotationSequenceAnglesUnits=deg  RotationMatrix=[1 0 0; 0 1 0; 0 0 1]  Quaternion=[1 0 0 0]
  Transform1 : sm_lib/Frames and Transforms/Rigid Transform  TranslationMethod=Cartesian  TranslationStandardOffset=0  TranslationLengthUnit=mm  TranslationStandardAxis=+Z  TranslationCartesianOffset=smiData.RigidTransform(7).translation  TranslationROffset=0  TranslationROffsetUnits=m  TranslationZOffset=0  TranslationZOffsetUnits=m  TranslationThetaOffset=0  TranslationThetaOffsetUnits=deg  RotationMethod=ArbitraryAxis  RotationAngleUnits=rad  RotationStandardAxis=+Z  RotationAngle=smiData.RigidTransform(7).angle  RotationArbitraryAxis=smiData.RigidTransform(7).axis  FollAlignAxisA=+X  BaseAlignAxisA=+Y  FollAlignAxisB=+Y  BaseAlignAxisB=+Z  RotationSequenceAxes=FollowerAxes  RotationSequence=XYX  RotationSequenceAngles=[0 0 0]  RotationSequenceAnglesUnits=deg  RotationMatrix=[1 0 0; 0 1 0; 0 0 1]  Quaternion=[1 0 0 0]
  Transform2 : sm_lib/Frames and Transforms/Rigid Transform  TranslationMethod=Cartesian  TranslationStandardOffset=0  TranslationLengthUnit=mm  TranslationStandardAxis=+Z  TranslationCartesianOffset=smiData.RigidTransform(9).translation  TranslationROffset=0  TranslationROffsetUnits=m  TranslationZOffset=0  TranslationZOffsetUnits=m  TranslationThetaOffset=0  TranslationThetaOffsetUnits=deg  RotationMethod=ArbitraryAxis  RotationAngleUnits=rad  RotationStandardAxis=+Z  RotationAngle=smiData.RigidTransform(9).angle  RotationArbitraryAxis=smiData.RigidTransform(9).axis  FollAlignAxisA=+X  BaseAlignAxisA=+Y  FollAlignAxisB=+Y  BaseAlignAxisB=+Z  RotationSequenceAxes=FollowerAxes  RotationSequence=XYX  RotationSequenceAngles=[0 0 0]  RotationSequenceAnglesUnits=deg  RotationMatrix=[1 0 0; 0 1 0; 0 0 1]  Quaternion=[1 0 0 0]
  Transform3 : sm_lib/Frames and Transforms/Rigid Transform  TranslationMethod=Cartesian  TranslationStandardOffset=0  TranslationLengthUnit=mm  TranslationStandardAxis=+Z  TranslationCartesianOffset=smiData.RigidTransform(11).translation  TranslationROffset=0  TranslationROffsetUnits=m  TranslationZOffset=0  TranslationZOffsetUnits=m  TranslationThetaOffset=0  TranslationThetaOffsetUnits=deg  RotationMethod=ArbitraryAxis  RotationAngleUnits=rad  RotationStandardAxis=+Z  RotationAngle=smiData.RigidTransform(11).angle  RotationArbitraryAxis=smiData.RigidTransform(11).axis  FollAlignAxisA=+X  BaseAlignAxisA=+Y  FollAlignAxisB=+Y  BaseAlignAxisB=+Z  RotationSequenceAxes=FollowerAxes  RotationSequence=XYX  RotationSequenceAngles=[0 0 0]  RotationSequenceAnglesUnits=deg  RotationMatrix=[1 0 0; 0 1 0; 0 0 1]  Quaternion=[1 0 0 0]
  Transform4 : sm_lib/Frames and Transforms/Rigid Transform  TranslationMethod=Cartesian  TranslationStandardOffset=0  TranslationLengthUnit=mm  TranslationStandardAxis=+Z  TranslationCartesianOffset=smiData.RigidTransform(13).translation  TranslationROffset=0  TranslationROffsetUnits=m  TranslationZOffset=0  TranslationZOffsetUnits=m  TranslationThetaOffset=0  TranslationThetaOffsetUnits=deg  RotationMethod=ArbitraryAxis  RotationAngleUnits=rad  RotationStandardAxis=+Z  RotationAngle=smiData.RigidTransform(13).angle  RotationArbitraryAxis=smiData.RigidTransform(13).axis  FollAlignAxisA=+X  BaseAlignAxisA=+Y  FollAlignAxisB=+Y  BaseAlignAxisB=+Z  RotationSequenceAxes=FollowerAxes  RotationSequence=XYX  RotationSequenceAngles=[0 0 0]  RotationSequenceAnglesUnits=deg  RotationMatrix=[1 0 0; 0 1 0; 0 0 1]  Quaternion=[1 0 0 0]
  Transform5 : sm_lib/Frames and Transforms/Rigid Transform  TranslationMethod=Cartesian  TranslationStandardOffset=0  TranslationLengthUnit=mm  TranslationStandardAxis=+Z  TranslationCartesianOffset=smiData.RigidTransform(15).translation  TranslationROffset=0  TranslationROffsetUnits=m  TranslationZOffset=0  TranslationZOffsetUnits=m  TranslationThetaOffset=0  TranslationThetaOffsetUnits=deg  RotationMethod=ArbitraryAxis  RotationAngleUnits=rad  RotationStandardAxis=+Z  RotationAngle=smiData.RigidTransform(15).angle  RotationArbitraryAxis=smiData.RigidTransform(15).axis  FollAlignAxisA=+X  BaseAlignAxisA=+Y  FollAlignAxisB=+Y  BaseAlignAxisB=+Z  RotationSequenceAxes=FollowerAxes  RotationSequence=XYX  RotationSequenceAngles=[0 0 0]  RotationSequenceAnglesUnits=deg  RotationMatrix=[1 0 0; 0 1 0; 0 0 1]  Quaternion=[1 0 0 0]
  Target : PMIOPort  Side=Left
  F5 : PMIOPort  Port=2  Side=Right
  F4 : PMIOPort  Port=3  Side=Right
  F2 : PMIOPort  Port=4  Side=Right
  F1 : PMIOPort  Port=5  Side=Right
  F : PMIOPort  Port=6  Side=Right
  connections:
  ReferenceFrame/RConn1 -- Transform/LConn1 -- Transform1/LConn1 -- Transform4/LConn1 -- Transform5/LConn1 -- Transform3/LConn1 -- Transform2/LConn1 -- Target/RConn1 -- Solid/RConn1
  Transform/RConn1 -- F/RConn1
  Transform1/RConn1 -- F1/RConn1
  Transform2/RConn1 -- F2/RConn1
  Transform4/RConn1 -- F4/RConn1
  Transform5/RConn1 -- F5/RConn1

== system minhUpdate/Steering System/Wheel Left/Innova_Crysta_Assembly_Final_1_RIGID ==
  Innova_Crysta_Rim_Design_attempt_1_1_RIGID : Subsystem
  Innova_Crysta_Tire_Design_Attempt_2_1_RIGID : Subsystem
  ReferenceFrame : sm_lib/Frames and Transforms/Reference Frame
  Transform : sm_lib/Frames and Transforms/Rigid Transform  TranslationMethod=Cartesian  TranslationStandardOffset=0  TranslationLengthUnit=mm  TranslationStandardAxis=+Z  TranslationCartesianOffset=smiData.RigidTransform(25).translation  TranslationROffset=0  TranslationROffsetUnits=m  TranslationZOffset=0  TranslationZOffsetUnits=m  TranslationThetaOffset=0  TranslationThetaOffsetUnits=deg  RotationMethod=ArbitraryAxis  RotationAngleUnits=rad  RotationStandardAxis=+Z  RotationAngle=smiData.RigidTransform(25).angle  RotationArbitraryAxis=smiData.RigidTransform(25).axis  FollAlignAxisA=+X  BaseAlignAxisA=+Y  FollAlignAxisB=+Y  BaseAlignAxisB=+Z  RotationSequenceAxes=FollowerAxes  RotationSequence=XYX  RotationSequenceAngles=[0 0 0]  RotationSequenceAnglesUnits=deg  RotationMatrix=[1 0 0; 0 1 0; 0 0 1]  Quaternion=[1 0 0 0]
  Transform1 : sm_lib/Frames and Transforms/Rigid Transform  TranslationMethod=Cartesian  TranslationStandardOffset=0  TranslationLengthUnit=mm  TranslationStandardAxis=+Z  TranslationCartesianOffset=smiData.RigidTransform(43).translation  TranslationROffset=0  TranslationROffsetUnits=m  TranslationZOffset=0  TranslationZOffsetUnits=m  TranslationThetaOffset=0  TranslationThetaOffsetUnits=deg  RotationMethod=ArbitraryAxis  RotationAngleUnits=rad  RotationStandardAxis=+Z  RotationAngle=smiData.RigidTransform(43).angle  RotationArbitraryAxis=smiData.RigidTransform(43).axis  FollAlignAxisA=+X  BaseAlignAxisA=+Y  FollAlignAxisB=+Y  BaseAlignAxisB=+Z  RotationSequenceAxes=FollowerAxes  RotationSequence=XYX  RotationSequenceAngles=[0 0 0]  RotationSequenceAnglesUnits=deg  RotationMatrix=[1 0 0; 0 1 0; 0 0 1]  Quaternion=[1 0 0 0]
  Transform2 : sm_lib/Frames and Transforms/Rigid Transform  TranslationMethod=Cartesian  TranslationStandardOffset=0  TranslationLengthUnit=mm  TranslationStandardAxis=+Z  TranslationCartesianOffset=smiData.RigidTransform(44).translation  TranslationROffset=0  TranslationROffsetUnits=m  TranslationZOffset=0  TranslationZOffsetUnits=m  TranslationThetaOffset=0  TranslationThetaOffsetUnits=deg  RotationMethod=ArbitraryAxis  RotationAngleUnits=rad  RotationStandardAxis=+Z  RotationAngle=smiData.RigidTransform(44).angle  RotationArbitraryAxis=smiData.RigidTransform(44).axis  FollAlignAxisA=+X  BaseAlignAxisA=+Y  FollAlignAxisB=+Y  BaseAlignAxisB=+Z  RotationSequenceAxes=FollowerAxes  RotationSequence=XYX  RotationSequenceAngles=[0 0 0]  RotationSequenceAnglesUnits=deg  RotationMatrix=[1 0 0; 0 1 0; 0 0 1]  Quaternion=[1 0 0 0]
  F : PMIOPort  Side=Right
  connections:
  Transform/LConn1 -- ReferenceFrame/RConn1 -- Transform1/LConn1 -- Transform2/LConn1
  Transform/RConn1 -- F/RConn1
  Innova_Crysta_Rim_Design_attempt_1_1_RIGID/LConn1 -- Transform1/RConn1
  Innova_Crysta_Tire_Design_Attempt_2_1_RIGID/LConn1 -- Transform2/RConn1
